simulink model "a_T_vector_tgo_iterator"  (R2016b)
settings: Solver=VariableStepAuto  StartTime=0.0  StopTime=100  RelTol=1e-3
values from neighbouring files (symbols this model uses):
  m0 = 58000    [E_Guidance_Modular.m]    (also in E_Guidance_Wong.m; E_Guidance_advanced.m; E_Guidance_advanced_hybrid.m; E_Guidance_advanced_thrust_optimization.m)
  mu = 4.282828185603917*10^13    (= 4.2828281856e+13)    [E_Guidance_Modular.m]    (also in E_Guidance_Wong.m; E_Guidance_advanced.m; E_Guidance_advanced_hybrid.m; E_Guidance_advanced_thrust_optimization.m)
  r0 = A*r0    [E_Guidance_Modular.m]    (also in E_Guidance_Wong.m; E_Guidance_advanced.m; E_Guidance_advanced_hybrid.m; E_Guidance_advanced_thrust_optimization.m)
  rf = A*rf    [E_Guidance_Modular.m]    (also in E_Guidance_Wong.m; E_Guidance_advanced.m; E_Guidance_advanced_hybrid.m; E_Guidance_advanced_thrust_optimization.m)
  T_max = 800000    [E_Guidance_Modular.m]    (also in E_Guidance_Wong.m; E_Guidance_advanced.m; E_Guidance_advanced_hybrid.m; E_Guidance_advanced_thrust_optimization.m)
  T_min = 200000    [E_Guidance_Modular.m]    (also in E_Guidance_Wong.m; E_Guidance_advanced.m; E_Guidance_advanced_hybrid.m; E_Guidance_advanced_thrust_optimization.m)
  tol_tgo = 0.01    [E_Guidance_sim.m]
  V0 = A*V0    [E_Guidance_Modular.m]    (also in E_Guidance_Wong.m; E_Guidance_advanced.m; E_Guidance_advanced_hybrid.m; E_Guidance_advanced_thrust_optimization.m)
  v_ex = 3531.7    [E_Guidance_Modular.m]    (also in E_Guidance_Wong.m; E_Guidance_advanced.m; E_Guidance_advanced_hybrid.m; E_Guidance_advanced_thrust_optimization.m)
  Vf = A*Vf    [E_Guidance_Modular.m]    (also in E_Guidance_Wong.m; E_Guidance_advanced.m; E_Guidance_advanced_hybrid.m; E_Guidance_advanced_thrust_optimization.m)
settings Model: Creator=lloyd.strohl  LastModifiedBy=lloyd.strohl

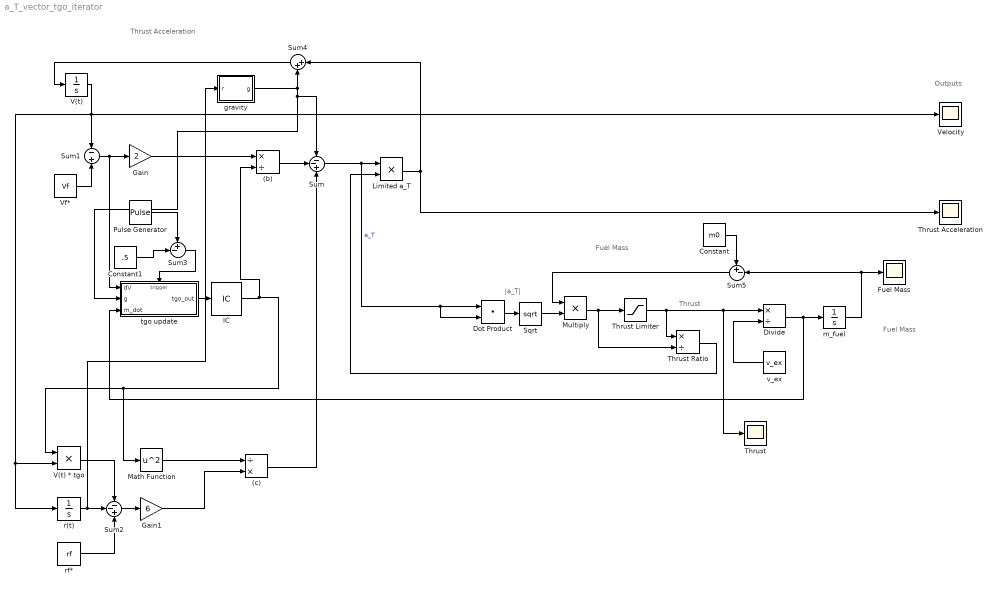
== system a_T_vector_tgo_iterator ==
  note: Fuel Mass
  note: Thrust
  note: Fuel Mass
  note: Outputs
  note: Thrust Acceleration
  note: |a_T|
  (b) : Product  Inputs=*/
  (c) : Product  Inputs=/*
  Constant : Constant  Value=m0
  Constant1 : Constant  Value=.5
  Divide : Product  Inputs=*/
  Dot Product : DotProduct  InputSameDT=on  OutDataTypeStr=Inherit: Inherit via internal rule
  Fuel Mass : Scope
  Gain : Gain  Gain=2
  Gain1 : Gain  Gain=6
  IC : InitialCondition  Value=60
  Limited a_T : Product  Inputs=**
  Math Function : Math  Operator=square  SaturateOnIntegerOverflow=on
  Multiply : Product
  Pulse Generator : DiscretePulseGenerator  PulseType=Time based  Period=10  PulseWidth=5
  Sqrt : Sqrt  SaturateOnIntegerOverflow=on
  Sum : Sum  Inputs=--+
  Sum1 : Sum  Inputs=-+
  Sum2 : Sum  Inputs=--+
  Sum3 : Sum  Inputs=+-|
  Sum4 : Sum  Inputs=|++
  Sum5 : Sum  Inputs=+-|
  Thrust : Scope
  Thrust Acceleration : Scope
  Thrust Limiter : Saturate  UpperLimit=T_max  LowerLimit=T_min
  Thrust Ratio : Product  Inputs=*/
  V(t) : Integrator  InitialCondition=V0  ContinuousStateAttributes='Velocity'
  V(t) * tgo : Product
  Velocity : Scope
  Vf* : Constant  Value=Vf
  gravity : Subsystem
  m_fuel : Integrator  ContinuousStateAttributes='Fuel_Mass'
  r(t) : Integrator  InitialCondition=r0  ContinuousStateAttributes='Position'
  rf* : Constant  Value=rf
  tgo update : Subsystem  TreatAsAtomicUnit=on
  v_ex : Constant  Value=v_ex
  wires:
  gravity/1(g) -> Sum4/2, tgo update/2(g), Sum/1
  r(t)/1 -> gravity/1(r), Sum2/2
  V(t)/1 -> Velocity/1, Sum1/1, V(t) * tgo/2, r(t)/1
  (b)/1 -> Sum/2
  Sum1/1 -> tgo update/1(dV), Gain/1
  Gain/1 -> (b)/1
  Sum2/1 -> Gain1/1
  Gain1/1 -> (c)/2
  Math Function/1 -> (c)/1
  (c)/1 -> Sum/3
  rf*/1 -> Sum2/3
  V(t) * tgo/1 -> Sum2/1
  Vf*/1 -> Sum1/2
  Sqrt/1 -> Multiply/2
  v_ex/1 -> Divide/2
  Divide/1 -> tgo update/3(m_dot), m_fuel/1
  m_fuel/1 -> Fuel Mass/1, Sum5/2
  Sum4/1 -> V(t)/1
  Sum5/1 -> Multiply/1
  Constant/1 -> Sum5/1
  Dot Product/1 -> Sqrt/1
  Multiply/1 -> Thrust Ratio/2, Thrust Limiter/1
  Thrust Limiter/1 -> Thrust Ratio/1, Divide/1, Thrust/1
  Sum/1 -> Dot Product/2, Dot Product/1, Limited a_T/1  "a_T"
  Thrust Ratio/1 -> Limited a_T/2
  Limited a_T/1 -> Sum4/1, Thrust Acceleration/1
  tgo update/1(tgo_out) -> IC/1
  IC/1 -> Math Function/1, V(t) * tgo/1, (b)/2
  Pulse Generator/1 -> Sum3/1
  Constant1/1 -> Sum3/2
  Sum3/1 -> tgo update/Trigger

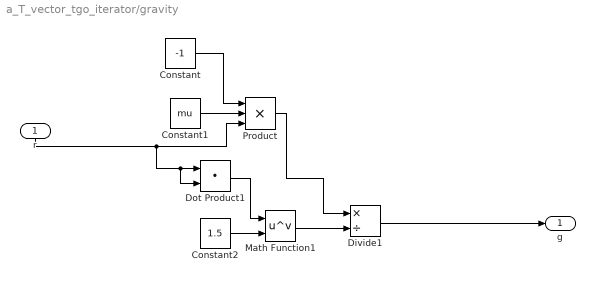
== system a_T_vector_tgo_iterator/gravity ==
  r : Inport
  Constant : Constant  Value=-1
  Constant1 : Constant  Value=mu
  Constant2 : Constant  Value=1.5
  Divide1 : Product  Inputs=*/
  Dot Product1 : DotProduct  InputSameDT=on  OutDataTypeStr=Inherit: Inherit via internal rule
  Math Function1 : Math  Operator=pow  SaturateOnIntegerOverflow=on
  Product : Product  Inputs=***
  g : Outport
  wires:
  r/1 -> Product/3, Dot Product1/2, Dot Product1/1
  Math Function1/1 -> Divide1/2
  Product/1 -> Divide1/1
  Constant2/1 -> Math Function1/2
  Dot Product1/1 -> Math Function1/1
  Divide1/1 -> g/1
  Constant1/1 -> Product/2
  Constant/1 -> Product/1

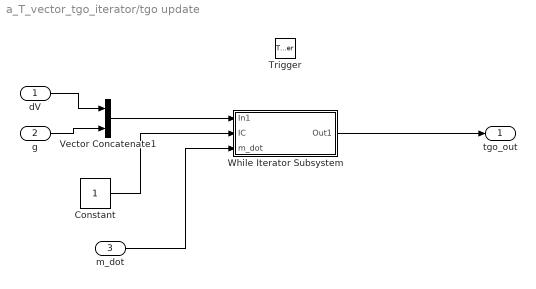
== system a_T_vector_tgo_iterator/tgo update ==
  dV : Inport
  g : Inport  Port=2
  m_dot : Inport  Port=3  LatchByDelayingOutsideSignal=on
  Trigger : TriggerPort  VariantControl=Variant
  Constant : Constant  OutDataTypeStr=boolean
  Vector Concatenate1 : Concatenate
  While Iterator Subsystem : Subsystem  TreatAsAtomicUnit=on
  tgo_out : Outport
  wires:
  dV/1 -> Vector Concatenate1/1
  g/1 -> Vector Concatenate1/2
  Vector Concatenate1/1 -> While Iterator Subsystem/1(In1)
  m_dot/1 -> While Iterator Subsystem/3(m_dot)
  Constant/1 -> While Iterator Subsystem/2(IC)
  While Iterator Subsystem/1(Out1) -> tgo_out/1

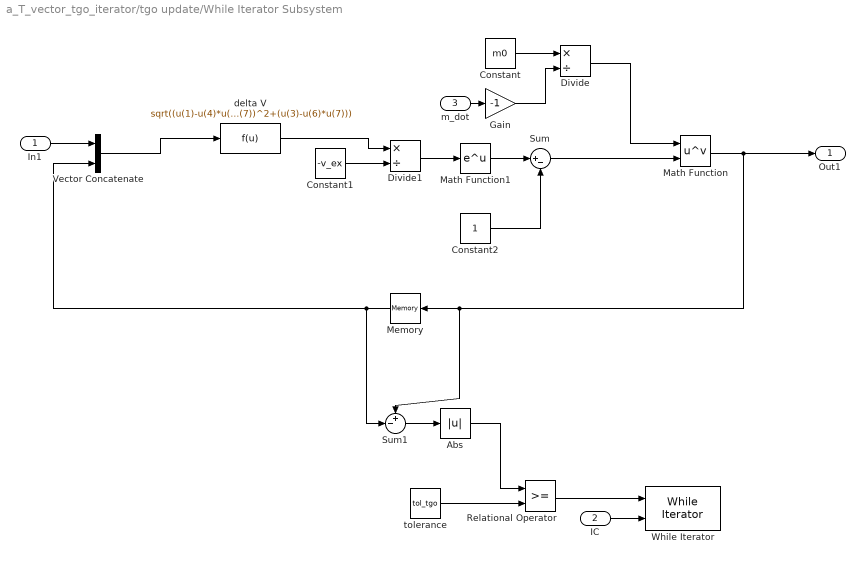
== system a_T_vector_tgo_iterator/tgo update/While Iterator Subsystem ==
  In1 : Inport
  IC : Inport  Port=2
  m_dot : Inport  Port=3
  Abs : Abs
  Constant : Constant  Value=m0
  Constant1 : Constant  Value=-v_ex
  Constant2 : Constant
  Divide : Product  Inputs=*/
  Divide1 : Product  Inputs=*/
  Gain : Gain  Gain=-1
  Math Function : Math  Operator=pow  SaturateOnIntegerOverflow=on
  Math Function1 : Math  SaturateOnIntegerOverflow=on
  Memory : Memory  X0=50  InheritSampleTime=on
  Relational Operator : RelationalOperator  OutDataTypeStr=boolean  RndMeth=Simplest
  Sum : Sum  Inputs=|+-
  Sum1 : Sum  Inputs=+-|
  Vector Concatenate : Concatenate
  While Iterator : WhileIterator  MaxIters=100
  delta V : Fcn  Expr=sqrt((u(1)-u(4)*u(7))^2+(u(2)-u(5)*u(7))^2+(u(3)-u(6)*u(7)))
  tolerance : Constant  Value=tol_tgo
  Out1 : Outport
  wires:
  IC/1 -> While Iterator/2
  Constant/1 -> Divide/1
  delta V/1 -> Divide1/1
  Constant1/1 -> Divide1/2
  Divide1/1 -> Math Function1/1
  Math Function1/1 -> Sum/1
  Constant2/1 -> Sum/2
  Divide/1 -> Math Function/1
  Sum/1 -> Math Function/2
  Math Function/1 -> Out1/1, Sum1/1, Memory/1
  m_dot/1 -> Gain/1
  Gain/1 -> Divide/2
  Vector Concatenate/1 -> delta V/1
  In1/1 -> Vector Concatenate/1
  Memory/1 -> Sum1/2, Vector Concatenate/2
  tolerance/1 -> Relational Operator/2
  Sum1/1 -> Abs/1
  Abs/1 -> Relational Operator/1
  Relational Operator/1 -> While Iterator/1
